simulink model "verify_Economy_Ecology_mdl"  (R2016b)
settings: Solver=ode45  StartTime=0  StopTime=24*3600+1  MaxStep=1800  RelTol=1e-3  EnableMultiTasking=on
libraries: carnot x3
settings Model: Creator=drhf  LastModifiedBy=drhf
settings DataIOCC: SaveFormat=Array  SignalLoggingSaveFormat=ModelDataLogs
settings OptimizationCC: ExpressionDepthLimit=2147483647  LifeSpan=inf
settings DebuggingCC: UnderspecifiedInitializationDetection=Classic  MergeDetectMultiDrivingBlocksExec=none  SolverPrmCheckMsg=warning  FcnCallInpInsideContextMsg=warning  StateNameClashWarn=warning  SFUnexpectedBacktrackingDiag=warning  SFNoUnconditionalDefaultTransitionDiag=warning  SFExecutionAtInitializationDiag=none
settings HardwareCC: ProdBitPerPointer=32  ProdBitPerSizeT=32  ProdBitPerPtrDiffT=32  ProdLargestAtomicFloat=None  ProdIntDivRoundTo=Undefined  ProdEndianess=Unspecified  ProdWordSize=32  ProdHWDeviceType=32-bit Generic
settings ModelReferenceCC: PropagateSignalLabelsOutOfModel=off
settings GRTTargetCC: TargetLangStandard=C89/C90 (ANSI)  GeneratePreprocessorConditionals=Disable all  CombineOutputUpdateFcns=off  GRTInterface=on
settings ConfigComp: CovMetricSettings=dw  CovHtmlReporting=on  CovSaveCumulativeToWorkspaceVar=on  CovSaveSingleToWorkspaceVar=on  CovExternalEMLEnable=off

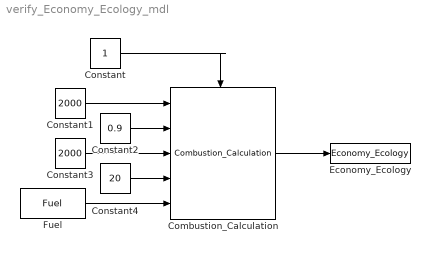
== system verify_Economy_Ecology_mdl ==
  Combustion_Calculation : carnot/Basic/Thermal_Models/Combustion_Calculation
  Constant : Constant
  Constant1 : Constant  Value=2000
  Constant2 : Constant  Value=0.9
  Constant3 : Constant  Value=2000
  Constant4 : Constant  Value=20
  Economy_Ecology : carnot/Toolbox/Economy_Ecology
  Fuel : carnot/Source/Energy/Fuel  ft=1  t=20  ls=3.5  p=1.013e5  h_values=[5.14e7 5.69e7]  tc=45  price=1  mass=[0.33 0.67 0 0 0 0]
  wires:
  Combustion_Calculation/1 -> Economy_Ecology/1
  Constant/1 -> Combustion_Calculation/Enable
  Constant1/1 -> Combustion_Calculation/1
  Constant2/1 -> Combustion_Calculation/2
  Constant3/1 -> Combustion_Calculation/3
  Constant4/1 -> Combustion_Calculation/4
  Fuel/1 -> Combustion_Calculation/5
